simulink model "V02_pendulum"  (R2018b)
settings: Solver=ode1  StartTime=0.0  StopTime=2  FixedStep=0.001  RelTol=1e-3
model workspace (MAT data in the model file):
  J = 2
  L = 0.5
  M = 3
  g = 9.81
settings Model: Creator=Administrator  LastModifiedBy=Administrator

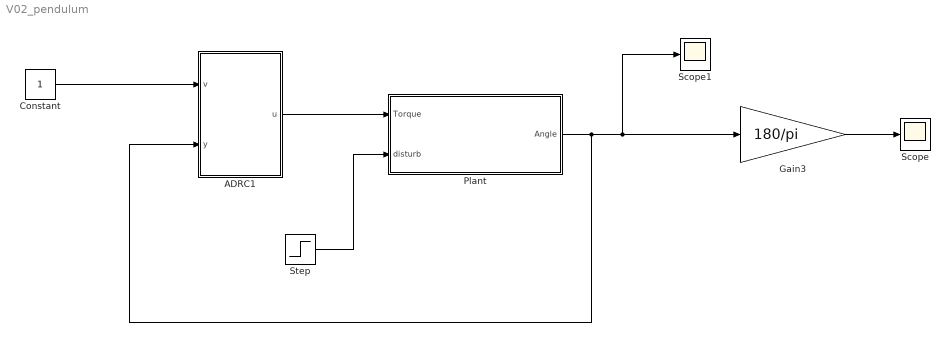
== system V02_pendulum ==
  ADRC1 : Subsystem
  Constant : Constant
  Gain3 : Gain  Gain=180/pi
  Plant : Subsystem
  Scope : Scope
  Scope1 : Scope
  Step : Step  After=600  SampleTime=0
  wires:
  Gain3/1 -> Scope/1
  Constant/1 -> ADRC1/1(v)
  Plant/1(Angle) -> ADRC1/2(y), Scope1/1, Gain3/1
  ADRC1/1(u) -> Plant/1(Torque)
  Step/1 -> Plant/2("disturb ")

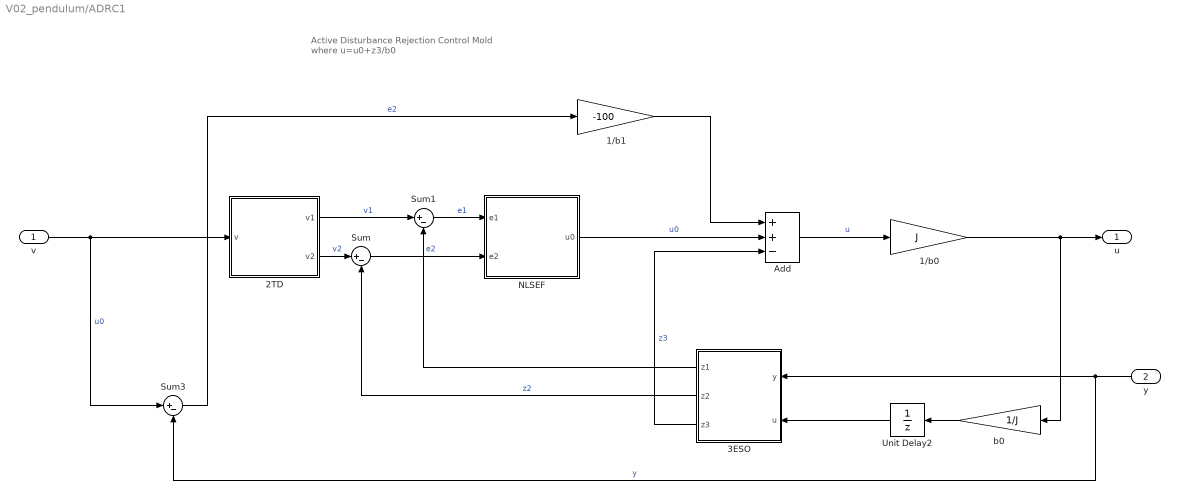
== system V02_pendulum/ADRC1 ==
  note: Active Disturbance Rejection Control Mold
      |
      | where u=u0+z3/b0
  v : Inport
  y : Inport  Port=2
  1/b0 : Gain  Gain=J
  1/b1 : Gain  Gain=-100
  2TD : Subsystem
  3ESO : Subsystem
  Add : Sum  Inputs=++-
  NLSEF : MATLAB Function  TreatAsAtomicUnit=on
  Sum : Sum  Inputs=|+-
  Sum1 : Sum  Inputs=|+-
  Sum3 : Sum  Inputs=|+-
  Unit Delay2 : UnitDelay  SampleTime=-1
  b0 : Gain  Gain=1/J
  u : Outport
  wires:
  Add/1 -> 1/b0/1  "u"
  y/1 -> Sum3/2, 3ESO/1(y)  "y"
  b0/1 -> Unit Delay2/1
  3ESO/3(z3) -> Add/3  "z3"
  3ESO/1(z1) -> Sum1/2
  3ESO/2(z2) -> Sum/2  "z2"
  1/b0/1 -> b0/1, u/1
  Sum1/1 -> NLSEF/1(e1)  "e1"
  Sum/1 -> NLSEF/2(e2)  "e2"
  2TD/2(v2) -> Sum/1  "v2"
  2TD/1(v1) -> Sum1/1  "v1"
  v/1 -> Sum3/1, 2TD/1(v)  "u0"
  Unit Delay2/1 -> 3ESO/2(u)
  NLSEF/1(u0) -> Add/2  "u0"
  1/b1/1 -> Add/1
  Sum3/1 -> 1/b1/1  "e2"

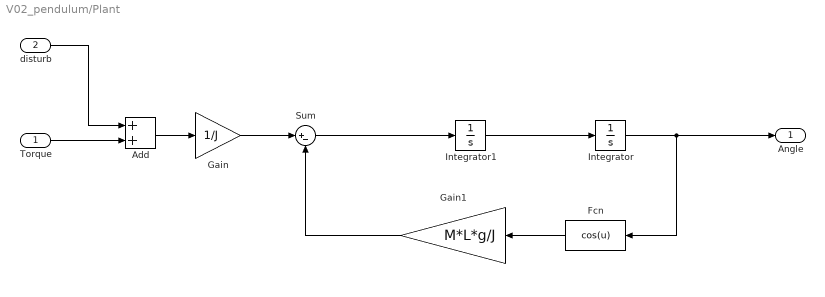
== system V02_pendulum/Plant ==
  Torque : Inport
  "disturb " : Inport  Port=2
  Add : Sum
  Fcn : Fcn  Expr=cos(u)
  Gain : Gain  Gain=1/J
  Gain1 : Gain  Gain=M*L*g/J
  Integrator : Integrator
  Integrator1 : Integrator
  Sum : Sum  Inputs=|+-
  Angle : Outport
  wires:
  Sum/1 -> Integrator1/1
  Gain1/1 -> Sum/2
  Fcn/1 -> Gain1/1
  Integrator1/1 -> Integrator/1
  Gain/1 -> Sum/1
  Integrator/1 -> Angle/1, Fcn/1
  Add/1 -> Gain/1
  Torque/1 -> Add/2
  "disturb "/1 -> Add/1

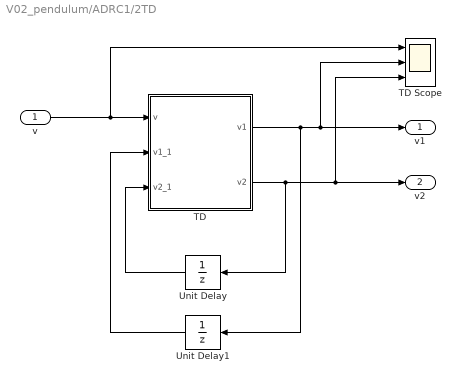
== system V02_pendulum/ADRC1/2TD ==
  v : Inport
  TD : MATLAB Function  TreatAsAtomicUnit=on
  TD Scope : Scope  NumInputPorts=3
  Unit Delay : UnitDelay  SampleTime=-1
  Unit Delay1 : UnitDelay  SampleTime=-1
  v1 : Outport
  v2 : Outport  Port=2
  wires:
  v/1 -> TD/1(v), TD Scope/1
  TD/1(v1) -> Unit Delay1/1, v1/1, TD Scope/2
  TD/2(v2) -> Unit Delay/1, v2/1, TD Scope/3
  Unit Delay/1 -> TD/3(v2_1)
  Unit Delay1/1 -> TD/2(v1_1)

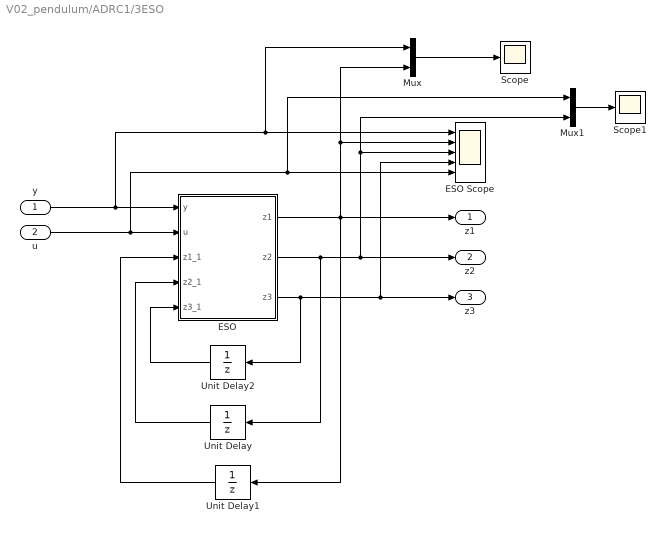
== system V02_pendulum/ADRC1/3ESO ==
  y : Inport
  u : Inport  Port=2
  ESO : MATLAB Function  TreatAsAtomicUnit=on
  ESO Scope : Scope  NumInputPorts=5
  Mux : Mux  Inputs=2
  Mux1 : Mux  Inputs=2
  Scope : Scope
  Scope1 : Scope
  Unit Delay : UnitDelay  SampleTime=-1
  Unit Delay1 : UnitDelay  SampleTime=-1
  Unit Delay2 : UnitDelay  SampleTime=-1
  z1 : Outport
  z2 : Outport  Port=2
  z3 : Outport  Port=3
  wires:
  Mux1/1 -> Scope1/1
  Mux/1 -> Scope/1
  u/1 -> ESO Scope/5, Mux1/1, ESO/2(u)
  y/1 -> ESO Scope/1, Mux/1, ESO/1(y)
  Unit Delay1/1 -> ESO/3(z1_1)
  Unit Delay/1 -> ESO/4(z2_1)
  Unit Delay2/1 -> ESO/5(z3_1)
  ESO/3(z3) -> ESO Scope/4, z3/1, Unit Delay2/1
  ESO/2(z2) -> ESO Scope/3, Mux1/2, z2/1, Unit Delay/1
  ESO/1(z1) -> ESO Scope/2, Mux/2, Unit Delay1/1, z1/1

== matlab function V02_pendulum/ADRC1/2TD/TD ==
  data: v input; v1 output; v1_1 input; v2_1 input; v2 output
function [v1,v2] = fcn(v, v1_1,v2_1)
% This block supports the Embedded MATLAB subset.
% See the help menu for details. 

%parameter
r=700;
h=0.001;
k=20;
h0=k*h;

%function fhan(vv1_1-v,v2_1,r,h0)
d=r*power(h0,2);
a0=h0*v2_1;
y=v1_1-v+a0;             
a1=power(d*(d+8*abs(y)),0.5);
a2=a0+sign(y)*(a1-d)/2;
sy=(sign(y+d)-sign(y-d))/2;
a=(a0+y-a2)*sy+a2;
sa=(sign(a+d)-sign(a-d))/2;
fhan=-r*(a/d-sign(a))*sa-r*sign(a);
fh=fhan;

%TD equation
v1=v1_1+h*v2_1;
v2=v2_1+h*fh;

== matlab function V02_pendulum/ADRC1/NLSEF ==
  data: e1 input; u0 output; e2 input
function u0 = fcn(e1,e2)
% This block supports the Embedded MATLAB subset.
% See the help menu for details. 

% %The first method:u0=k1*fal1(e1,alpha1,delta)+k2*fal2(e2,alpha2,delta)
% %0<alpha1<1<alpha2
% % %parameter
% alpha1=0.2;
% alpha2=1.1;
% delta=0.5;
% k1=5;
% k2=1;
% s1 = (sign(e1+delta)-sign(e1-delta))/2;
% s2 = (sign(e2+delta)-sign(e2-delta))/2;
% fal1 = e1*s1/power(delta,(1-alpha1)) + power(abs(e1),alpha1)*sign(e1)*(1-s1);
% fal2 = e2*s2/power(delta,(1-alpha2)) + power(abs(e2),alpha2)*sign(e2)*(1-s2);
% fe = fal1; fe1 = fal2;
% %NLSEF equation
% u0=k1*fe+k2*fe1;

%The second method:u0=-fhan(e1,ce2,r,h1)
%parameter
% c=0.3;%原来的参数
% r=5;
% h1=0.001;
c=1; %c一般指的是阻尼系数，一般取1，这样处于临界阻尼状态
r=500;%r越大，收敛越快
h1=0.005;%通常h1是步长的20~5倍之间,r取较大值时会出现超调，适当减小h1值，会使得超调减小。
%function fhan(vv1_1-v,v2_1,r,h0)
d=r*power(h1,2);
a0=h1*c*e2;
y=e1+a0;             
a1=power(d*(d+8*abs(y)),0.5);
a2=a0+sign(y)*(a1-d)/2;
sy=(sign(y+d)-sign(y-d))/2;
a=(a0+y-a2)*sy+a2;
sa=(sign(a+d)-sign(a-d))/2;
fhan=-r*(a/d-sign(a))*sa-r*sign(a);

u0=-fhan;

%The third method:u0=k1*e1+k2*e2;
%parameter
% k1=10;
% k2=1;
% u0=k1*e1+k2*e2;

== matlab function V02_pendulum/ADRC1/3ESO/ESO ==
  data: y input; u input; z1_1 input; z2_1 input; z3_1 input; z1 output; z2 output; z3 output
function [z1,z2,z3] = fcn(y,u,z1_1,z2_1,z3_1)
% This block supports the Embedded MATLAB subset.
% See the help menu for details. 

%parameter
h = 0.001;
% k=1;
k=10;
delta = k*h;
beta01 = 1/h;
beta02 = 1/(1.6*power(h,1.5));
beta03 = 1/(8.6*power(h,2.2));
% beta01 = 1/h;
% beta02 = 1/(3*power(h,2));
% beta03 = 1/(20*power(h,3));
% beta01 = 1/h;
% beta02 = 1/(3*power(h,2));
% beta03 = 1/(power(8,2)*power(h,3));
% beta01 = 300;
% beta02 = 1500;
% beta03 = 200;

e=z1_1-y;

s = (sign(e+delta)-sign(e-delta))/2;
fal1 = e*s/power(delta,(1-0.5)) + power(abs(e),0.5)*sign(e)*(1-s);
fal2 = e*s/power(delta,(1-0.25)) + power(abs(e),0.25)*sign(e)*(1-s);
fe = fal1; fe1 = fal2;

%ESO equation
z1 = z1_1 + h*(z2_1-beta01*e);
z2 = z2_1 + h*(z3_1-beta02*fe + u);
z3 = z3_1 + h*(-beta03*fe1);
